simulink model "SteeringEffortModel"  (R2020a)
settings: Solver=VariableStepAuto  StartTime=0.0  StopTime=10  RelTol=1e-3
undefined symbols (not defined in the file or in its folder): Col, Joint, Rack
libraries: simulink x1
settings Model: Creator=lopez  LastModifiedBy=eggsy
settings SFSimCC: CustomCodeUndefinedFunction=UseInterfaceOnly

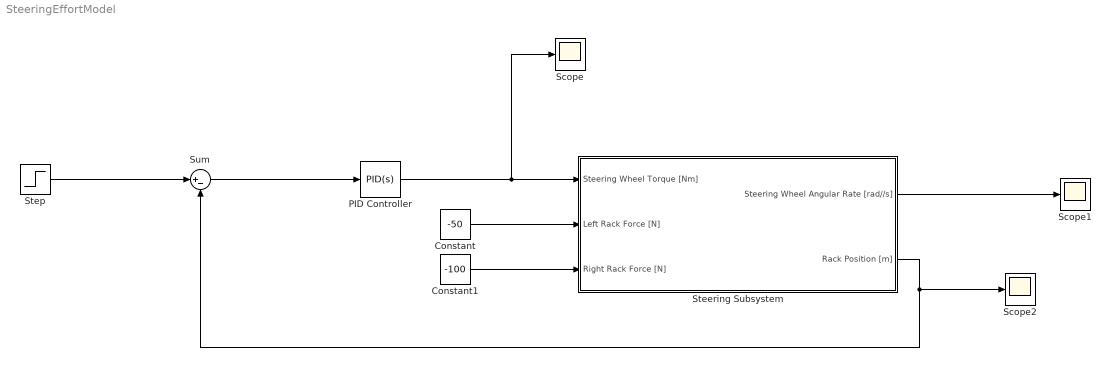
== system SteeringEffortModel ==
  Constant : Constant  Value=-50
  Constant1 : Constant  Value=-100
  PID Controller : simulink/Continuous/PID Controller  Controller=PID  Form=Ideal  TimeDomain=Continuous-time  UseExternalTs=off  SampleTime=-1  IntegratorMethod=Forward Euler  FilterMethod=Forward Euler  ControllerParametersSource=internal  P=4  I=2  D=5  UseFilter=on  N=100  TunerSelectOption=Transfer Function Based (PID Tuner App)  InitialConditionSource=internal  InitialConditionForIntegrator=0  InitialConditionForFilter=0  DifferentiatorICPrevScaledInput=0  ExternalReset=none  TrackingMode=off  Kt=1  LimitOutput=on  UpperSaturationLimit=7  LowerSaturationLimit=-7  LinearizeAsGain=on  AntiWindupMode=none  Kb=1  POutMin=[]  POutMax=[]  IOutMin=[]  IOutMax=[]  DOutMin=[]  DOutMax=[]  NOutMin=[]  NOutMax=[]  SumOutMin=[]  SumOutMax=[]  SaturationOutMin=[]  SaturationOutMax=[]  PParamMin=[]  PParamMax=[]  IParamMin=[]  IParamMax=[]  DParamMin=[]  DParamMax=[]  NParamMin=[]  NParamMax=[]  KbParamMin=[]  KbParamMax=[]  KtParamMin=[]  KtParamMax=[]  KbOutMin=[]  KbOutMax=[]  KtOutMin=[]  KtOutMax=[]  IntegratorOutMin=[]  IntegratorOutMax=[]  FilterOutMin=[]  FilterOutMax=[]  SumI1OutMin=[]  SumI1OutMax=[]  SumI2OutMin=[]  SumI2OutMax=[]  SumI3OutMin=[]  SumI3OutMax=[]  SumI4OutMin=[]  SumI4OutMax=[]  SumDOutMin=[]  SumDOutMax=[]  DifferentiatorOutMin=[]  DifferentiatorOutMax=[]  FilterDiffOutCoefMin=[]  FilterDiffOutCoefMax=[]  ReciprocalOutMin=[]  ReciprocalOutMax=[]  SumDenOutMin=[]  SumDenOutMax=[]  SumNumOutMin=[]  SumNumOutMax=[]  DivideOutMin=[]  DivideOutMax=[]  UdiffTsProdOutMin=[]  UdiffTsProdOutMax=[]  NTsProdOutMin=[]  NTsProdOutMax=[]  UintegralTsProdOutMin=[]  UintegralTsProdOutMax=[]  UngainTsProdOutMin=[]  UngainTsProdOutMax=[]  IntegratorContinuousStateAttributes=''  IntegratorStateMustResolveToSignalObject=off  IntegratorRTWStateStorageClass=Auto  FilterContinuousStateAttributes=''  FilterStateMustResolveToSignalObject=off  FilterRTWStateStorageClass=Auto  ParallelPVariant=Passthrough  IdealPVariant=InternalParameters  IVariant=InternalParameters  DVariant=InternalParameters  IntegratorVariant=Continuous  SatVariant=Enabled  AWVariant=Passthrough  PCopyVariant=Disabled  TRVariant=Disabled  FdbkBlocksVariant=Forward  IdealPFdbkVariant=Disabled  SatFdbkVariant=Disabled  DerivativeFilterVariant=ContFilter  NVariant=InternalParameters  NCopyVariant=Disabled  FilterICVariant=InternalICsFilter  IntegratorICVariant=InternalICs  ExternalResetVariant=Disabled  TRSumVariant=Passthrough  SumFdbkVariant=Disabled  SumVariant=Sum_PID  TsampFilterVariant=InternalTs  TsampNgainVariant=Passthrough  TsampIntegralVariant=Passthrough
  Scope : Scope
  Scope1 : Scope
  Scope2 : Scope
  Steering Subsystem : Subsystem
  Step : Step  After=0.01  SampleTime=0
  Sum : Sum  Inputs=|+-
  wires:
  PID Controller/1 -> Scope/1, Steering Subsystem/1(Steering Wheel Torque [Nm])
  Sum/1 -> PID Controller/1
  Steering Subsystem/2(Rack Position [m]) -> Scope2/1, Sum/2
  Constant/1 -> Steering Subsystem/2(Left Rack Force [N])
  Steering Subsystem/1(Steering Wheel Angular Rate [rad//s]) -> Scope1/1
  Step/1 -> Sum/1
  Constant1/1 -> Steering Subsystem/3(Right Rack Force [N])

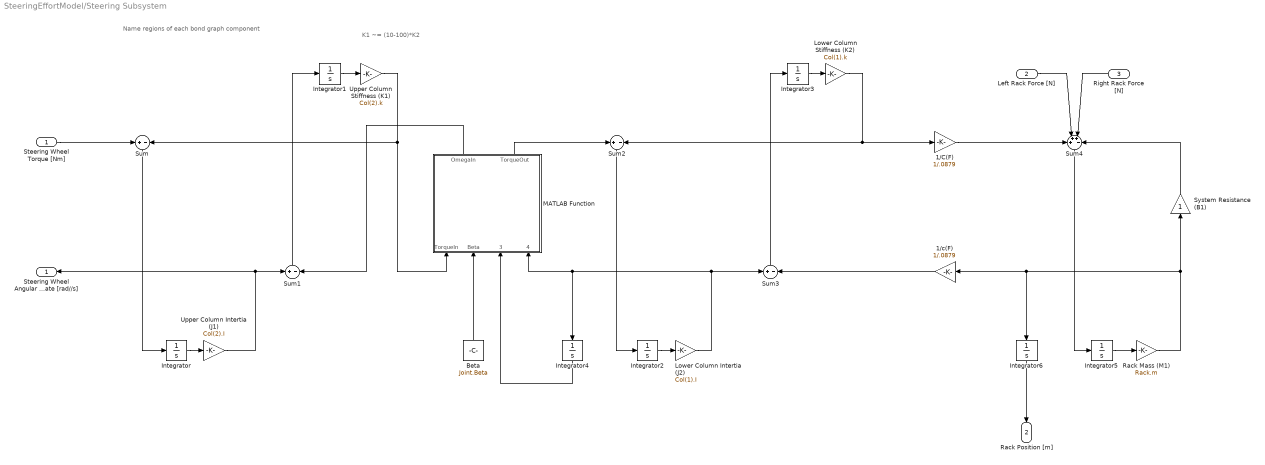
== system SteeringEffortModel/Steering Subsystem ==
  note: K1 ~= (10-100)*K2
  note: Name regions of each bond graph component
  Steering Wheel Torque [Nm] : Inport  OutMin=[135]
  Left Rack Force [N] : Inport  Port=2
  Right Rack Force [N] : Inport  Port=3
  1/C(F) : Gain  Gain=1/.0879
  1/c(F) : Gain  Gain=1/.0879
  Beta : Constant  Value=Joint.Beta
  Integrator{,1..6} (7 alike) : Integrator
  Lower Column Intertia (J2) : Gain  Gain=Col(1).I
  Lower Column Stiffness (K2) : Gain  Gain=Col(1).k
  MATLAB Function : MATLAB Function  TreatAsAtomicUnit=on
  Rack Mass (M1) : Gain  Gain=Rack.m
  Sum{,1..3} (4 alike) : Sum  Inputs=+-
  Sum4 : Sum  Inputs=+++-
  System Resistance (B1) : Gain
  Upper Column Intertia (J1) : Gain  Gain=Col(2).I
  Upper Column Stiffness (K1) : Gain  Gain=Col(2).k
  Steering Wheel Angular Rate [rad//s] : Outport
  Rack Position [m] : Outport  Port=2
  wires:
  Lower Column Stiffness (K2)/1 -> 1/C(F)/1, Sum2/2
  1/c(F)/1 -> Sum3/2
  Integrator4/1 -> MATLAB Function/3(ThetaOut)
  Integrator5/1 -> Rack Mass (M1)/1
  Upper Column Stiffness (K1)/1 -> MATLAB Function/1(TorqueIn), Sum/2
  Sum/1 -> Integrator/1
  MATLAB Function/2(TorqueOut) -> Sum2/1
  Rack Mass (M1)/1 -> System Resistance (B1)/1, Integrator6/1, 1/c(F)/1
  Integrator2/1 -> Lower Column Intertia (J2)/1
  Sum3/1 -> Integrator3/1
  Sum2/1 -> Integrator2/1
  Beta/1 -> MATLAB Function/2(Beta)
  Integrator/1 -> Upper Column Intertia (J1)/1
  MATLAB Function/1(OmegaIn) -> Sum1/2
  Upper Column Intertia (J1)/1 -> Steering Wheel Angular Rate [rad//s]/1, Sum1/1
  Integrator3/1 -> Lower Column Stiffness (K2)/1
  Sum1/1 -> Integrator1/1
  1/C(F)/1 -> Sum4/1
  Sum4/1 -> Integrator5/1
  Integrator1/1 -> Upper Column Stiffness (K1)/1
  Lower Column Intertia (J2)/1 -> MATLAB Function/4(OmegaOut), Integrator4/1, Sum3/1
  Steering Wheel Torque [Nm]/1 -> Sum/1
  System Resistance (B1)/1 -> Sum4/4
  Right Rack Force [N]/1 -> Sum4/3
  Left Rack Force [N]/1 -> Sum4/2
  Integrator6/1 -> Rack Position [m]/1

== matlab function SteeringEffortModel/Steering Subsystem/MATLAB Function ==
  data: TorqueIn input; Beta input; ThetaOut input; OmegaIn output; TorqueOut output; OmegaOut input
function [OmegaIn, TorqueOut] = CardenTransformation(TorqueIn,Beta,ThetaOut,OmegaOut)

OmegaIn = OmegaOut .* cosd(Beta) ./ ( 1 - (sind(Beta).*cos(ThetaOut)).^2 );

TorqueOut = TorqueIn .* cosd(Beta) ./ ( 1 - (sind(Beta).*cos(ThetaOut)).^2 );
